simulink model "qpsk_demo"  (R2016a)
settings: Solver=VariableStepDiscrete  SolverMode=SingleTasking  StartTime=0.0  StopTime=3e6  RelTol=1e-3
PreLoadFcn:
  | load('sdrqpskrx.mat')
  | load('sdrqpsktx.mat')
  | load data_Yb
  | DataIn = Yb_with_time(:,2);
  | WL=14;
  | n = length(DataIn);
undefined symbols (not defined in the file): dfilt, gcbh, rcfiltgaincompat, sdrqpskrx, sdrqpsktx
libraries: dspobslib x3, commfilt2 x2, commrfcorlib x1, commrflib2 x1, commblksprivate x1, dspspect3 x1, commutil2 x1, dspbuff3 x1, commrandsrc2 x1, commdigbbndpm3 x1
settings Model: Creator=mdonovan  LastModifiedBy=lenovo
settings DataIOCC: LimitDataPoints=on  SaveFormat=Array  SignalLoggingSaveFormat=ModelDataLogs  SaveOutput=off  SignalLogging=off  SaveTime=off
settings OptimizationCC: BlockReduction=off  BooleanDataType=off  ConditionallyExecuteInputs=off  DefaultParameterBehavior=Inlined  ExpressionDepthLimit=2147483647  LocalBlockOutputs=off
settings DebuggingCC: AlgebraicLoopMsg=error  UnderspecifiedInitializationDetection=Classic  MergeDetectMultiDrivingBlocksExec=none  SolverPrmCheckMsg=warning  SingleTaskRateTransMsg=error  FcnCallInpInsideContextMsg=UseLocalSettings  StateNameClashWarn=warning
settings HardwareCC: ProdBitPerPointer=32  ProdLargestAtomicFloat=None  ProdIntDivRoundTo=Undefined  ProdEndianess=Unspecified  ProdWordSize=32  ProdHWDeviceType=32-bit Generic
settings ModelReferenceCC: PropagateSignalLabelsOutOfModel=off
settings GRTTargetCC: CombineOutputUpdateFcns=off  GRTInterface=on
settings ConfigComp: CovModelRefEnable=Off  CovSFcnEnable=off

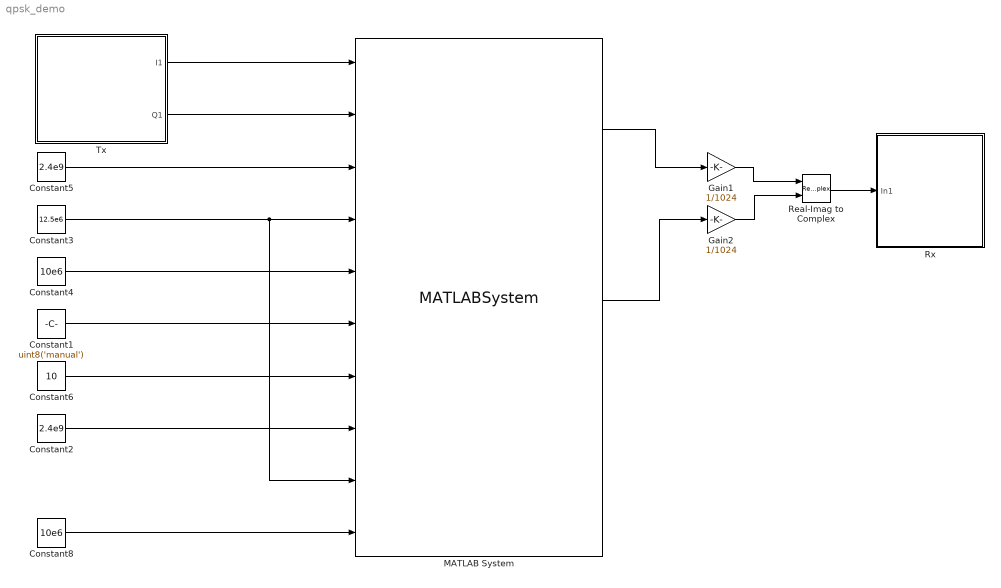
== system qpsk_demo ==
  Constant1 : Constant  Value=uint8('manual')  SampleTime=-1
  Constant2 : Constant  Value=2.4e9  SampleTime=-1
  Constant3 : Constant  Value=12.5e6  SampleTime=-1
  Constant4 : Constant  Value=10e6  SampleTime=-1
  Constant5 : Constant  Value=2.4e9  SampleTime=-1
  Constant6 : Constant  Value=10  SampleTime=-1
  Constant8 : Constant  Value=10e6  SampleTime=-1
  Gain1 : Gain  Gain=1/1024
  Gain2 : Gain  Gain=1/1024
  MATLAB System : MATLABSystem  DialogController=sysobjdialog.BlockDynDialog  System=iio_sys_obj  ip_address=192.168.2.1  dev_name=ad9361  in_ch_no=2  in_ch_size=240000  out_ch_no=2  out_ch_size=240000  SimulateUsing=Interpreted execution
      mask Type: iio_sys_obj
      mask Display:
      | disp('ad9361');
      | port_label('input',1,'DATA_IN1');
      | port_label('input',2,'DATA_IN2');
      | port_label('input',3,'RX_LO_FREQ');
      | port_label('input',4,'RX_SAMPLING_FREQ');
      | port_label('input',5,'RX_RF_BANDWIDTH');
      | port_label('input',6,'RX1_GAIN_MODE');
      | port_label('input',7,'RX1_GAIN');
      | port_label('input',8,'TX_LO_FREQ');
      | port_label('input',9,'TX_SAMPLING_FREQ');
      | port_label('input',10,'TX_RF_BANDWIDTH');
      | port_label('output',1,'DATA_OUT1');
      | port_label('output',2,'DATA_OUT2');
      | port_label('output',3,'RX1_RSSI');
  Real-Imag to Complex : RealImagToComplex
  Rx : Subsystem
  Tx : Subsystem
  wires:
  MATLAB System/1 -> Gain1/1
  MATLAB System/2 -> Gain2/1
  Constant5/1 -> MATLAB System/3
  Constant3/1 -> MATLAB System/9, MATLAB System/4
  Constant4/1 -> MATLAB System/5
  Constant1/1 -> MATLAB System/6
  Constant8/1 -> MATLAB System/10
  Gain1/1 -> Real-Imag to Complex/1
  Gain2/1 -> Real-Imag to Complex/2
  Tx/1(I1) -> MATLAB System/1
  Tx/2(Q1) -> MATLAB System/2
  Real-Imag to Complex/1 -> Rx/1(In1)
  Constant2/1 -> MATLAB System/8
  Constant6/1 -> MATLAB System/7

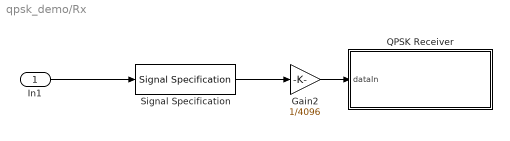
== system qpsk_demo/Rx ==
  In1 : Inport
  Gain2 : Gain  Gain=1/4096
  QPSK Receiver : Subsystem
      mask Display: disp('QPSK Receiver')
  Signal Specification : SignalSpecification  SampleTime=sdrqpskrx.RadioFrameSize/sdrqpskrx.Fs
  wires:
  Gain2/1 -> QPSK Receiver/1(dataIn)
  In1/1 -> Signal Specification/1
  Signal Specification/1 -> Gain2/1

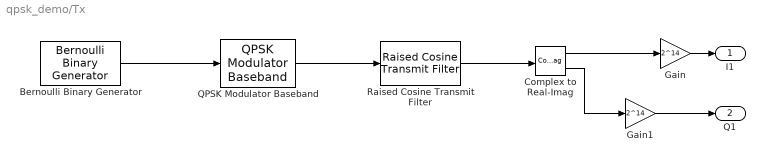
== system qpsk_demo/Tx ==
  Bernoulli Binary Generator : commrandsrc2/Bernoulli Binary Generator  P=0.5  seed=61  Ts=-1  frameBased=on  sampPerFrame=120000  orient=off  outDataType=double
  Complex to Real-Imag : ComplexToRealImag
  Gain : Gain  Gain=2^14
  Gain1 : Gain  Gain=2^14
  QPSK Modulator Baseband : commdigbbndpm3/QPSK Modulator Baseband  InType=Bit  Enc=Gray  Ph=pi/4  outDtype=double  outWordLen=16  outUDDataType=sfix(16)  outFracLenMode=Best precision  outFracLen=15  outDataTypeStr=double  outLastDataTypeStr=double
  Raised Cosine Transmit Filter : commfilt2/Raised Cosine Transmit Filter  filtType=Square root  R=0.5  filtSpan=2*((sdrqpsktx.RCFiltSpan)/2)  N=sdrqpsktx.Upsampling  filterGain=rcfiltgaincompat(gcbh)  InputProcessing=Columns as channels (frame based)  RateOptions=Enforce single-rate processing  framing=Mute  checkCoeff=off  variableName=rcTxFilt1  checkGain=Normalized  sampMode=Mute  saveAsFlag=0  currentFiltSpan=2*((sdrqpsktx.RCFiltSpan)/2)  D=(sdrqpsktx.RCFiltSpan)/2  launchFVT=off  roundingMode=Floor  overflowMode=off  coeffDataTypeStr=Inherit: Same word length as input  coeffMin=[]  coeffMax=[]  coeffLastDataTypeStr=Inherit: Same word length as input  outputDataTypeStr=Inherit: Same as accumulator  outputMin=[]  outputMax=[]  outputLastDataTypeStr=Inherit: Same as accumulator
  I1 : Outport
  Q1 : Outport  Port=2
  wires:
  Gain1/1 -> Q1/1
  Gain/1 -> I1/1
  Bernoulli Binary Generator/1 -> QPSK Modulator Baseband/1
  QPSK Modulator Baseband/1 -> Raised Cosine Transmit Filter/1
  Raised Cosine Transmit Filter/1 -> Complex to Real-Imag/1
  Complex to Real-Imag/2 -> Gain1/1
  Complex to Real-Imag/1 -> Gain/1

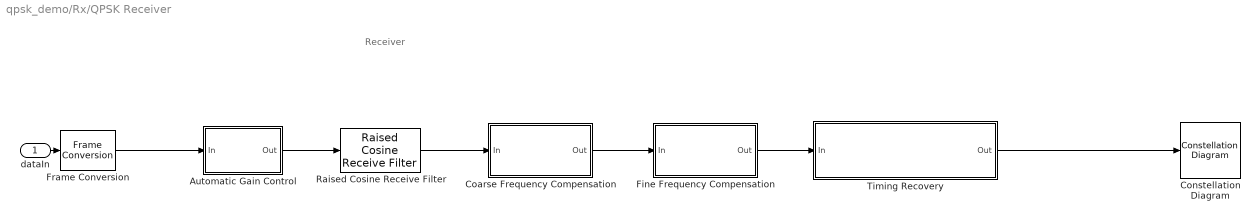
== system qpsk_demo/Rx/QPSK Receiver ==
  note: Receiver
  dataIn : Inport
  Automatic Gain Control : Subsystem  mask{DesiredAmplitude=1/sqrt(sdrqpskrx.Upsampling)}
      mask prompts: DesiredAmplitude "Desired Amplitude"
      mask Display: disp('Automatic Gain\nControl')
  Coarse Frequency Compensation : Subsystem
      mask Display: disp('Coarse Frequency\nCompensation');
  Constellation Diagram : ConstellationDiagram
  Fine Frequency Compensation : Subsystem
      mask Display: disp('Fine Frequency\nCompensation')
  Frame Conversion : FrameConversion  InheritSamplingMode=off
  Raised Cosine Receive Filter : commfilt2/Raised Cosine Receive Filter  filtType=Square root  R=0.5  filtSpan=2*((sdrqpskrx.RCFiltSpan)/2)  N=sdrqpskrx.Upsampling  downFactor=sdrqpskrx.Downsampling  downOffset=0  filterGain=rcfiltgaincompat(gcbh)  InputProcessing=Columns as channels (frame based)  RateOptions=Enforce single-rate processing  framing=Mute  checkCoeff=off  variableName=rcRxFilt1  currentFiltSpan=2*((sdrqpskrx.RCFiltSpan)/2)  D=(sdrqpskrx.RCFiltSpan)/2  inputOffset=0  sampMode=Mute  saveAsFlag=0  rateMode=Downsampling  checkGain=Normalized  launchFVT=off  roundingMode=Floor  overflowMode=off  coeffDataTypeStr=Inherit: Same word length as input  coeffMin=[]  coeffMax=[]  coeffLastDataTypeStr=Inherit: Same word length as input  accumDataTypeStr=Inherit: Same as product output  accumLastDataTypeStr=Inherit: Same as product output  outputDataTypeStr=Inherit: Same as accumulator  outputMin=[]  outputMax=[]  outputLastDataTypeStr=Inherit: Same as accumulator
  Timing Recovery : Subsystem
      mask Display:
      | disp('Timing\nRecovery');
      | port_label('output',1,'DataOut');
      | port_label('output',2,'DataValid');
  wires:
  Fine Frequency Compensation/1(Out) -> Timing Recovery/1(In)
  dataIn/1 -> Frame Conversion/1
  Timing Recovery/1(Out) -> Constellation Diagram/1
  Raised Cosine Receive Filter/1 -> Coarse Frequency Compensation/1(In)
  Coarse Frequency Compensation/1(Out) -> Fine Frequency Compensation/1(In)
  Frame Conversion/1 -> Automatic Gain Control/1(In)
  Automatic Gain Control/1(Out) -> Raised Cosine Receive Filter/1

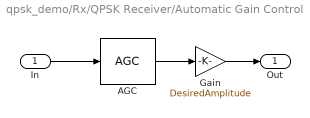
== system qpsk_demo/Rx/QPSK Receiver/Automatic Gain Control ==
  In : Inport
  AGC : commrfcorlib/AGC  LegacyMode=off  DetectorMethod=Rectifier  LoopMethod=Linear  UpdatePeriod=40  StepSize=0.1  AdaptationStepSize=(0.1)/(40)  DesiredOutputPower=1  AveragingLength=40  MaximumGain=1e6  MaxPowerGain=2*(1e6)  GainOutputPort=off  InputPowerOutputPort=off  SimulateUsing=Interpreted execution
  Gain : Gain  Gain=DesiredAmplitude
  Out : Outport
  wires:
  In/1 -> AGC/1
  AGC/1 -> Gain/1
  Gain/1 -> Out/1

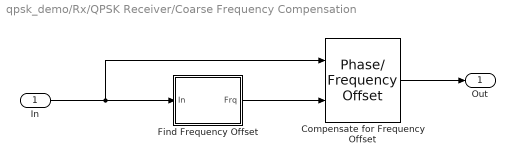
== system qpsk_demo/Rx/QPSK Receiver/Coarse Frequency Compensation ==
  In : Inport
  Compensate for Frequency Offset : commrflib2/Phase// Frequency Offset  phaseOffset=0  freqPort=on  freqOffset=100
  Find Frequency Offset : Subsystem  mask(Find Frequency Offset){M=sdrqpskrx.M, fftLen=1024, fftAvgs=32}
      mask prompts: M "Modulation order (integer):"; fftLen "FFT length (integer):"; fftAvgs "FFT averages (integer):"
  Out : Outport
  wires:
  In/1 -> Compensate for Frequency Offset/1, Find Frequency Offset/1(In)
  Compensate for Frequency Offset/1 -> Out/1
  Find Frequency Offset/1(Frq) -> Compensate for Frequency Offset/2

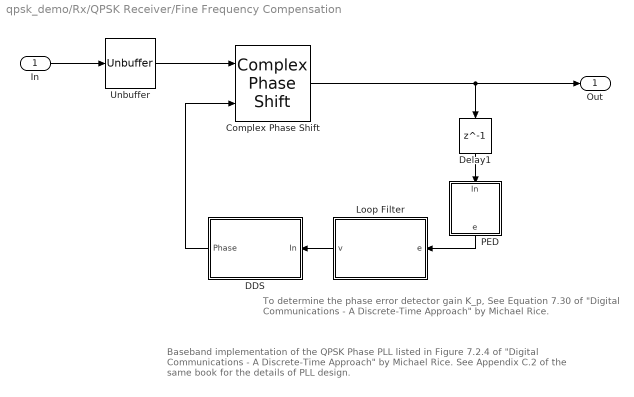
== system qpsk_demo/Rx/QPSK Receiver/Fine Frequency Compensation ==
  note: To determine the phase error detector gain K_p, See Equation 7.30 of "Digital
      | Communications - A Discrete-Time Approach" by Michael Rice.
  note: Baseband implementation of the QPSK Phase PLL listed in Figure 7.2.4 of
      | "Digital Communications - A Discrete-Time Approach" by Michael Rice. See
      | Appendix C.2 of the same book for the details of PLL design.
  In : Inport
  Complex Phase Shift : commutil2/Complex Phase Shift
  DDS : Subsystem
      mask Display: disp('DDS')
  Delay1 : Delay  DelayLength=1  InitialCondition=0  InputProcessing=Columns as channels (frame based)
  Loop Filter : Subsystem  mask{BnTs=0.06, zeta=2, N=sdrqpskrx.Upsampling/sdrqpskrx.Downsampling, Kp=sdrqpskrx.FineFreqPEDGain, K0=sdrqpskrx.FineFreqCompensateGain}
      mask prompts: BnTs "Normalized Loop Bandwidth"; zeta "Damping Factor"; N "Number of Samples/Symbol"; Kp "Phase Detector Gain (Kp)"; K0 "DDS Gain (K0)"
      mask init:
      | % See C.57 to C.61 in Michael Rice's "Digital Communications 
      | % - A Discrete-Time Approach" for details
      | theta = BnTs/(zeta+0.25/zeta)/N;
      | d = 1 + 2*zeta*theta + theta*theta;
      | K1 = 4*zeta*theta/d;
      | K2 = 4*theta*theta/d;
      | K1 = K1/(Kp*K0);
      | K2 = K2/(Kp*K0);
      mask Display: disp('Loop Filter')
  PED : MATLAB Function  TreatAsAtomicUnit=on
  Unbuffer : Unbuffer  SampleBasedProcessing=Same as frame based
  Out : Outport
  wires:
  PED/1(e) -> Loop Filter/1(e)
  Loop Filter/1(v) -> DDS/1(In)
  DDS/1(Phase) -> Complex Phase Shift/2
  Unbuffer/1 -> Complex Phase Shift/1
  In/1 -> Unbuffer/1
  Complex Phase Shift/1 -> Delay1/1, Out/1
  Delay1/1 -> PED/1(In)

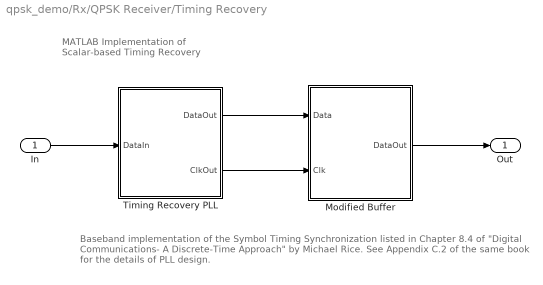
== system qpsk_demo/Rx/QPSK Receiver/Timing Recovery ==
  note: Baseband implementation of the Symbol Timing Synchronization listed in Chapter 8.4
      | of "Digital Communications- A Discrete-Time Approach" by Michael Rice. See
      | Appendix C.2 of the same book for the details of PLL design.
  note: MATLAB Implementation
      | of Scalar-based Timing Recovery
  In : Inport
  Modified Buffer : Subsystem  TreatAsAtomicUnit=on  mask(Input-Driven Buffer){bufSize=sdrqpskrx.FrameSize}
      mask prompts: bufSize "Buffer size:"
      mask help: A modified buffer subsystem that is driven by the arrival of its input data; it produces a valid output data buffer whenever its buffer is full and sets its dataValid flag to 1. Otherwise, the data at its dataOut port is not valid and its dataValid flag is set to 0.
  Timing Recovery PLL : Subsystem
      mask Display:
      | disp('Timing Recovery\nPLL')
      | port_label('input',1,'In')
      | port_label('output',1,'DataOut')
      | port_label('output',2,'Clk')
  Out : Outport
  wires:
  Timing Recovery PLL/2(ClkOut) -> Modified Buffer/2(Clk)
  Timing Recovery PLL/1(DataOut) -> Modified Buffer/1(Data)
  In/1 -> Timing Recovery PLL/1(DataIn)
  Modified Buffer/1(DataOut) -> Out/1

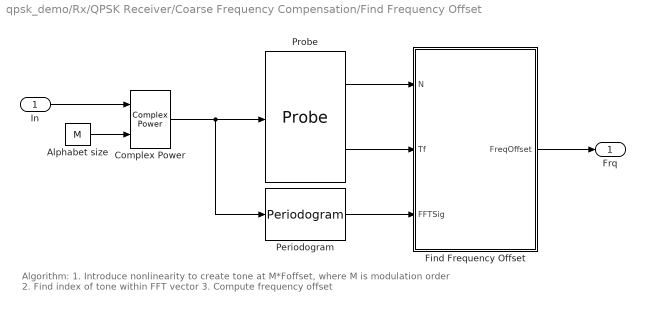
== system qpsk_demo/Rx/QPSK Receiver/Coarse Frequency Compensation/Find Frequency Offset ==
  note: Algorithm:
      | 1.  Introduce nonlinearity to create tone at M*Foffset, where M is modulation order
      | 2.  Find index of tone within FFT vector
      | 3.  Compute frequency offset
  In : Inport
  Alphabet size : Constant  Value=M  OutDataTypeStr=Inherit: Inherit via back propagation
  Complex Power : commblksprivate/Complex Power
  Find Frequency Offset : MATLAB Function  TreatAsAtomicUnit=on
  Periodogram : dspspect3/Periodogram  measurement=Power spectral density  wintype=Hamming  Rs=50  beta=5  winsamp=Symmetric  FFTImplementation=Auto  inheritFFT=off  fftsize=2048  navg=16  inheritTs=on  Ts=1
  Probe : Probe  ProbeComplexSignal=off
  Frq : Outport
  wires:
  Periodogram/1 -> Find Frequency Offset/3(FFTSig)
  Alphabet size/1 -> Complex Power/2
  In/1 -> Complex Power/1
  Probe/1 -> Find Frequency Offset/1(N)
  Probe/2 -> Find Frequency Offset/2(Tf)
  Find Frequency Offset/1(FreqOffset) -> Frq/1
  Complex Power/1 -> Probe/1, Periodogram/1

== system qpsk_demo/Rx/QPSK Receiver/Fine Frequency Compensation/DDS ==
  note: The digital filter acts as a pure integrator
  In : Inport
  Digital Filter : dspobslib/Digital Filter  TypePopup=IIR (poles & zeros)  IIRFiltStruct=Direct form II transposed  AllPoleFiltStruct=Direct form  FIRFiltStruct=Direct form  CoeffSource=Specify via dialog  NumCoeffs=[0 1]  DenCoeffs=[1 -1]  BiQuadCoeffs=[1 0.3 0.4 1 0.1 0.2]  LatticeCoeffs=[0.2 0.4]  denIgnore=on  FiltPerSampPopup=One filter per frame  IC=0  ICnum=0  ICden=0  roundingMode=Floor  overflowMode=off  ScaleValues=1  scaleValueFracLength=14  stageInFracLength=15  stageOutFracLength=15  FilterSource=Specify via dialog  dfiltObjectName=dfilt.dffir([1 2 1])  InputProcessing=Columns as channels (frame based)
  Gain : Gain  Gain=-1*sdrqpskrx.FineFreqCompensateGain
  Phase : Outport
  wires:
  Digital Filter/1 -> Gain/1
  In/1 -> Digital Filter/1
  Gain/1 -> Phase/1

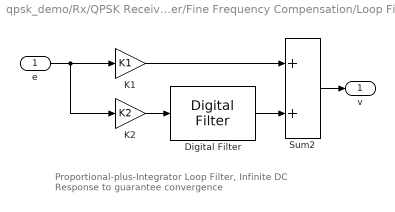
== system qpsk_demo/Rx/QPSK Receiver/Fine Frequency Compensation/Loop Filter ==
  note: Proportional-plus-Integrator Loop Filter,
      | Infinite DC Response to guarantee convergence
  e : Inport
  Digital Filter : dspobslib/Digital Filter  TypePopup=IIR (poles & zeros)  IIRFiltStruct=Direct form II transposed  AllPoleFiltStruct=Direct form  FIRFiltStruct=Direct form  CoeffSource=Specify via dialog  NumCoeffs=[1 0]  DenCoeffs=[1 -1]  BiQuadCoeffs=[1 0.3 0.4 1 0.1 0.2]  LatticeCoeffs=[0.2 0.4]  denIgnore=on  FiltPerSampPopup=One filter per frame  IC=0  ICnum=0  ICden=0  roundingMode=Floor  overflowMode=off  ScaleValues=1  scaleValueFracLength=14  stageInFracLength=15  stageOutFracLength=15  FilterSource=Specify via dialog  dfiltObjectName=dfilt.dffir([1 2 1])  InputProcessing=Columns as channels (frame based)
  K1 : Gain  Gain=K1
  K2 : Gain  Gain=K2
  Sum2 : Sum  SaturateOnIntegerOverflow=on  InputSameDT=on  OutDataTypeStr=Inherit: Same as first input
  v : Outport
  wires:
  K2/1 -> Digital Filter/1
  Digital Filter/1 -> Sum2/2
  Sum2/1 -> v/1
  e/1 -> K2/1, K1/1
  K1/1 -> Sum2/1

== system qpsk_demo/Rx/QPSK Receiver/Timing Recovery/Modified Buffer ==
  Data : Inport
  Clk : Inport  Port=2
  Modified Buffer : Subsystem
  DataOut : Outport
  wires:
  Data/1 -> Modified Buffer/1(In1)
  Clk/1 -> Modified Buffer/Enable
  Modified Buffer/1(DataOut) -> DataOut/1

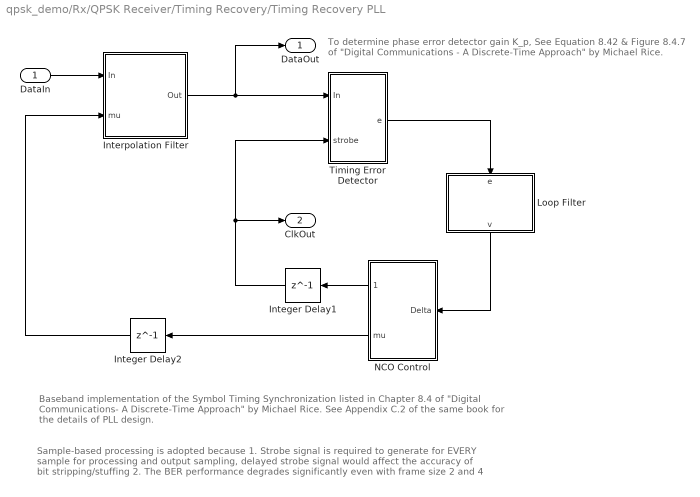
== system qpsk_demo/Rx/QPSK Receiver/Timing Recovery/Timing Recovery PLL ==
  note: Sample-based processing is adopted because
      | 1. Strobe signal is required to generate for EVERY sample for processing and output
      | sampling, delayed strobe signal would affect the accuracy of bit stripping/stuffing
      | 2. The BER performance degrades significantly even with frame size 2 and 4
  note: Baseband implementation of the Symbol Timing Synchronization listed in Chapter 8.4
      | of "Digital Communications- A Discrete-Time Approach" by Michael Rice. See Appendix
      | C.2 of the same book for the details of PLL design.
  note: To determine phase error detector gain K_p, See Equation 8.42 &
      | Figure 8.4.7 of "Digital Communications - A Discrete-Time Approach"
      | by Michael Rice.
  DataIn : Inport
  Integer Delay1 : Delay  DelayLength=1  InputProcessing=Inherited
  Integer Delay2 : Delay  DelayLength=1  InputProcessing=Inherited
  Interpolation Filter : MATLAB Function  TreatAsAtomicUnit=on
  Loop Filter : Subsystem  mask{BnTs=0.01, zeta=10, Kp=sdrqpskrx.TimingRecTEDGain, K0=sdrqpskrx.TimingRecCompensateGain, N=sdrqpskrx.Upsampling/sdrqpskrx.Downsampling}
      mask prompts: BnTs "Loop Bandwidth"; zeta "Loop Damping Factor"; Kp "Phase Detector Gain (Kp)"; K0 "DDS gain (K0)"; N "Number of Samples/symbol (N)"
      mask init:
      | % See C.57 to C.61 in Michael Rice's "Digital Communications 
      | % - A Discrete-Time Approach" for details
      | theta = BnTs/(zeta+0.25/zeta)/N;
      | d = 1 + 2*zeta*theta + theta*theta;
      | K1 = 4*zeta*theta/d;
      | K2 = 4*theta*theta/d;
      | K1 = K1/(Kp*K0);
      | K2 = K2/(Kp*K0);
      mask Display: disp('Loop Filter');
  NCO Control : MATLAB Function
  Timing Error Detector : MATLAB Function  TreatAsAtomicUnit=on
  DataOut : Outport
  ClkOut : Outport  Port=2
  wires:
  DataIn/1 -> Interpolation Filter/1(In)
  NCO Control/2(mu) -> Integer Delay2/1
  Integer Delay1/1 -> ClkOut/1, Timing Error Detector/2(strobe)
  NCO Control/1(Underflow) -> Integer Delay1/1
  Interpolation Filter/1(Out) -> DataOut/1, Timing Error Detector/1(In)
  Loop Filter/1(v) -> NCO Control/1(Delta)
  Timing Error Detector/1(e) -> Loop Filter/1(e)
  Integer Delay2/1 -> Interpolation Filter/2(mu)

== system qpsk_demo/Rx/QPSK Receiver/Timing Recovery/Modified Buffer/Modified Buffer ==
  In1 : Inport
  Enable : EnablePort
  Delay Line : dspbuff3/Delay Line  siz=bufSize  ic=0  directfeed=on  enable_output=off  hold_output=off  TreatMby1Signals=One channel  OutputFrames=on
  DataOut : Outport
  wires:
  Delay Line/1 -> DataOut/1
  In1/1 -> Delay Line/1

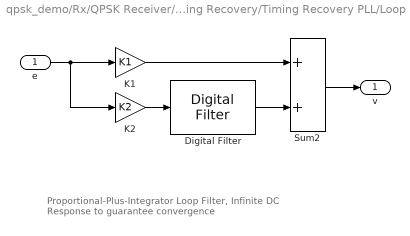
== system qpsk_demo/Rx/QPSK Receiver/Timing Recovery/Timing Recovery PLL/Loop Filter ==
  note: Proportional-Plus-Integrator Loop Filter,
      | Infinite DC Response to guarantee convergence
  e : Inport
  Digital Filter : dspobslib/Digital Filter  TypePopup=IIR (poles & zeros)  IIRFiltStruct=Direct form II transposed  AllPoleFiltStruct=Direct form  FIRFiltStruct=Direct form  CoeffSource=Specify via dialog  NumCoeffs=[1 0]  DenCoeffs=[1 -1]  BiQuadCoeffs=[1 0.3 0.4 1 0.1 0.2]  LatticeCoeffs=[0.2 0.4]  denIgnore=on  FiltPerSampPopup=One filter per frame  IC=0  ICnum=0  ICden=0  roundingMode=Floor  overflowMode=off  ScaleValues=1  scaleValueFracLength=14  stageInFracLength=15  stageOutFracLength=15  FilterSource=Specify via dialog  dfiltObjectName=dfilt.dffir([1 2 1])  InputProcessing=Columns as channels (frame based)
  K1 : Gain  Gain=K1
  K2 : Gain  Gain=K2
  Sum2 : Sum  SaturateOnIntegerOverflow=on  InputSameDT=on  OutDataTypeStr=Inherit: Same as first input
  v : Outport
  wires:
  K2/1 -> Digital Filter/1
  Digital Filter/1 -> Sum2/2
  Sum2/1 -> v/1
  e/1 -> K2/1, K1/1
  K1/1 -> Sum2/1

== matlab function qpsk_demo/Rx/QPSK Receiver/Coarse Frequency Compensation/Find Frequency Offset/Find Frequency Offset ==
  data: N input; FreqOffset output; Tf input; FFTSig input; M parameter
function FreqOffset = findfreqoffset(N,Tf,FFTSig,M) %#codegen
%  Estimate frequency offset.
%  findfreqoffset(N,Tf,fvec,params) returns the estimated frequency offset
%  given time-domain frame length N, sample time vector Tf containing
%  [frameTime,offsetTime], complex FFT vector FFTsig, and modulation
%  order M.

% Find index of max magnitude, convert to offset symmetric about zero.
% Return a negative integer offset to be interpreted as a compensation.
[~,maxIdx] = max(FFTSig);
FFTSize = size(FFTSig,1);
if maxIdx > FFTSize/2
    OffsetIdx = FFTSize+1-maxIdx;
else
    OffsetIdx = 1-maxIdx;
end
% Map offset index to a frequency value.
% Compute offset using modulation alphabet size params.M.
Ts = Tf(1)/N; % Sample time
delta_f = 1/(Ts*FFTSize); % Frequency resolution of FFT
FreqOffset = OffsetIdx * delta_f / M;

== matlab function qpsk_demo/Rx/QPSK Receiver/Fine Frequency Compensation/PED ==
  data: In input; e output
function e = PED(In)
% Implementation of Maximum Likelihood Phase Error Detector listed in
% Chapter 7.2.2 of "Digital Communications - A Discrete-Time Approach" by
% Michael Rice. This employs a decision directed method.
% 
% Input: 
%   In - Input samples, oversampled by two
% Output:
%   e - Phase error, de
%#codegen

e = sign(real(In)).*imag(In) - sign(imag(In)).*real(In);

== matlab function qpsk_demo/Rx/QPSK Receiver/Timing Recovery/Timing Recovery PLL/Interpolation Filter ==
  data: In input; Out output; mu input
function Out = interp_filter(In, mu)
% Prabolic piecewise polynomial interpolator, Farrow Interpolator with 
% alpha = 1/2, see Figure 8.4.16 of "Digital Communications - A 
% Discrete-Time Approach" by Michael Rice.
% Input:
%   In - Input samples, oversampled by two
%   mu - Difference between actual sampling instant and the optimal instant,
%        between zero and one
% Output:
%   Out - Interpolation output
%#codegen
persistent delay1 delay2 delay3; % Input delayed by 1, 2 and 3 samples
if isempty(delay1)
    [delay1, delay2, delay3] = deal(complex(0,0));
end

K = -0.5;

Out = delay2 + mu.*(K.*(In+delay2+delay3)+(1-K).*delay1)...
      + K.*(delay1+delay2-In-delay3).*mu.^2;
  
% Update delay buffers
delay3 = delay2;
delay2 = delay1;
delay1 = In;

== matlab function qpsk_demo/Rx/QPSK Receiver/Timing Recovery/Timing Recovery PLL/NCO Control ==
  data: Delta input; Underflow output; mu output; sdrqpskrx parameter
function [Underflow, mu] = NCO_ctrl(Delta, sdrqpskrx)
% Implementation of modulo-1 counter for interpolation control listed in
% Figure 8.4.19 of "Digital Communications - A Discrete-Time Approach"
% by Michael Rice. See design details in Chapter 8.4.3 of the same book.
% 
% Input:
%   Delta - Loop filter output. If loop is in lock, delta would be small
%   qpsktxrx - Simulation parameter structure
% Output:
%   Underflow - Indicator of counter underflow. This is the strobe signal
%   for downstream processing
%   mu - Difference between actual sampling instant and the optimal instant,
%        between zero and one
%#codegen

% delay1 - Counter value delayed by 1 sample
% Regtemp - The estimated timing error normalized by half QPSK symbols
persistent delay1 Regtemp;  
if isempty(delay1)
    [delay1, Regtemp] = deal(0);
end
Upsampling = sdrqpskrx.Upsampling;
Downsampling = sdrqpskrx.Downsampling;
oversampling = Upsampling/Downsampling;

counter = mod(delay1,1)-Delta-1/oversampling; % decrementing counter
if counter < 0
    Underflow = 1;
    Regtemp = mod(delay1,1)/(Delta+1/oversampling);
else
    Underflow = 0;
end

mu = Regtemp;

% Update delay buffer
delay1 = mod(delay1,1)-Delta-1/oversampling;

== matlab function qpsk_demo/Rx/QPSK Receiver/Timing Recovery/Timing Recovery PLL/Timing Error Detector ==
  data: In input; e output; strobe input
function e = TED(In, strobe)
% Zero-Crossing Timing Error Detector. See "Zero-Crossing Timing Error
% Detector" section in Chapter 8.4.1 of "Digital Communications - A
% Discrete-Time Approach" by Michael Rice. For bit stuffing/stripping
% details, see page 490-494 of the same book.
%
% Input: 
%   In - Input samples, interpolation result
%   strobe - Signal to enable timing error calculation
% Output:
%   e - Timing error
%#codegen
persistent delay1 delay2 delayStrobe; % Input delayed by one and 2 samples, and
% Enable signal delayed by one sample
if isempty(delay1)
    [delay1, delay2] = deal(complex(0,0));
    delayStrobe = 0;
end

if strobe==1 && delayStrobe~=strobe
    e = real(delay1) * (sign(real(delay2)) - sign(real(In))) + ...
        imag(delay1) * (sign(imag(delay2)) - sign(imag(In)));
else
    e = 0;
end

if delayStrobe~=strobe
    % Shift contents in delay register
    delay2 = delay1;
    delay1 = In;
elseif strobe==1
    % Two consecutive high strobes
    delay2 = 0; % Stuff missing sample
    delay1 = In; 
end
% If both current and previous enable signals are 0, skip current sample
% and keep the delayed signals unchanged. (Bit stripping)
delayStrobe = strobe;
